simulink model "Idealized_BB_Model"  (R2017a)
settings: Solver=VariableStepDiscrete  StartTime=0.0  StopTime=inf  FixedStep=1/(PSF_SampPerSym*Rsymbol*2)  RelTol=1e-3  EnableMultiTasking=on
PreLoadFcn:
  | %Rates
  | BitRate=(250)*1e3;
  | ChipRate=2e6;
  | SymRate=ChipRate/2;
  | RX_ChipDelay=6;
  | 
  | %Pulse shaping filter
  | OS=32;
  | 
  | Pin=-40;
  | 
  | Gain=45;
  | NF=9;
  | 
  | fc_RF=2450e6;
InitFcn:
  | x=linspace(0,1,OS);
  | weights=sin(pi*x);
libraries: dspmlti4 x2, dspmathops x2, commdigbbndpm3 x2, dspstat3 x2, commrandsrc2 x1, commseqgen2 x1, commfilt2 x1, commsink2 x1, rfmathmodels1 x1, simulink x1
settings Model: Creator=The MathWorks Inc.  LastModifiedBy=gzucchel
settings DataIOCC: LimitDataPoints=on  SaveFormat=Array  SignalLoggingSaveFormat=ModelDataLogs  SaveOutput=off  SignalLogging=off  DSMLogging=off  SaveTime=off
settings OptimizationCC: ExpressionDepthLimit=2147483647  LifeSpan=inf
settings DebuggingCC: UnderspecifiedInitializationDetection=Classic  MergeDetectMultiDrivingBlocksExec=none  SolverPrmCheckMsg=warning  FcnCallInpInsideContextMsg=warning  StateNameClashWarn=warning  SFUnexpectedBacktrackingDiag=warning  SFNoUnconditionalDefaultTransitionDiag=warning  SFExecutionAtInitializationDiag=none
settings HardwareCC: ProdBitPerPointer=32  ProdBitPerSizeT=32  ProdBitPerPtrDiffT=32  ProdLargestAtomicFloat=None  ProdIntDivRoundTo=Undefined  ProdEndianess=Unspecified  ProdWordSize=32  ProdHWDeviceType=32-bit Generic
settings ModelReferenceCC: PropagateSignalLabelsOutOfModel=off
settings GRTTargetCC: TargetLangStandard=C89/C90 (ANSI)  GeneratePreprocessorConditionals=Disable all  CombineOutputUpdateFcns=off  GRTInterface=on
settings ConfigComp: CovMetricSettings=dw  CovHtmlReporting=on  CovSaveCumulativeToWorkspaceVar=on  CovSaveSingleToWorkspaceVar=on  CovExternalEMLEnable=off  CovSFcnEnable=off
settings SimscapeCC: SimscapeNormalizeSystem=off  SimscapeNominalValues="[{\"value\":\"10\",\"unit\":\"V\"},{\"value\":\"1\",\"unit\":\"A\"},{\"value\":\"10\",\"unit\":\"N*m\"},{\"value\":\"10\",\"unit\":\"bar\"},{\"value\":\"100\",\"unit\":\"kJ/kg\"},{\"value\":\"1\",\"unit\":\"kW\"},{\"value\":\"300\",\"unit\":\"K\"},{\"value\":\"100\",\"unit\":\"cm^3/s\"},{\"value\":\"1\",\"unit\":\"kN\"},{\"value\":\"1\",\"unit\":\"g/cm^3\"},{\"value\":\"1\",\"unit\":\"l\"},{\"value\":\"1\",\"unit\":\"cm^2\"},{\"value\":\"60\",\"unit\":\"Hz\"}]"
settings ConfigurationSet: Description=SimMechanics 2G

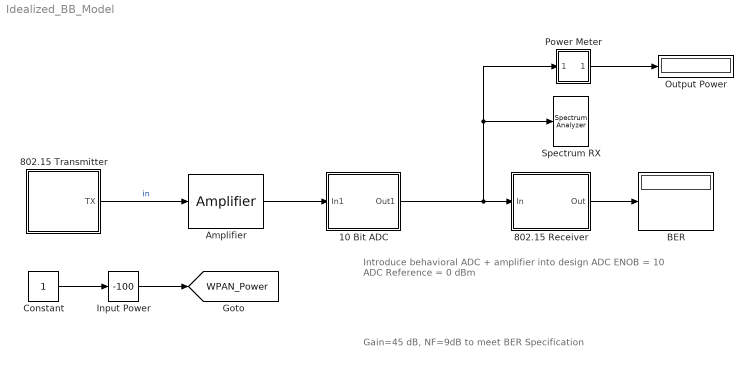
== system Idealized_BB_Model ==
  note: Introduce behavioral ADC + amplifier into design
      | ADC ENOB = 10
      | ADC Reference = 0 dBm
  note: Gain=45 dB, NF=9dB to meet BER Specification
  10 Bit ADC : Subsystem  mask{FS_P_dBm=0, Rnorm=1, N=10, Sample_Rate=0.0}
      mask prompts: FS_P_dBm "Full Scale Power"; Rnorm "Normalization Resistance"; Sample_Rate "Sample Rate (-1 for inherited)"
      mask init:
      | %LSB=FS_V/(2^(N-1));
      | %MAX=FS_V-LSB;
      | %MIN=-FS_V+LSB;
      | LSB=sqrt(2*Rnorm)*sqrt(1e-3)*sqrt(10^(FS_P_dBm/10))/(2^(N-1));
      | MAXp=sqrt(2*Rnorm)*sqrt(1e-3)*sqrt(10^(FS_P_dBm/10))-LSB;
      | MINp=-sqrt(2*Rnorm)*sqrt(1e-3)*sqrt(10^(FS_P_dBm/10))+LSB;
  802.15 Transmitter : Subsystem
  802.15 Receiver : Subsystem
  Amplifier : rfmathmodels1/Amplifier  model_select=Linear  linGaindB=Gain  GindB=0  iip3=30  am2pm=10  PwrAMPMStart=10  PwrAMPMEnd=inf  amam=[2.1587 1.1517]  ampm=[4.0033 9.1040]  x=[8.1081 1.5413 6.5202 -0.0718]  y=[4.6645 2.0965 10.88 -0.003]  p=0.5  GoutdB=0  vsat=1  method_select=Noise figure  ntemp=290  nfigure=NF  nfactor=0  seed=67987
      settings: SourceProductName=RF Toolbox  SourceProductBaseCode=RF
  BER : Display
  Constant : Constant
  Input Power : simulink/Math Operations/Slider Gain  gain=-100  low=-120  high=-30
  Output Power : Display
  Power Meter : Subsystem  mask{R=1, PB=off, buffer_sz=32*32}
      mask prompts: R "Resistance"; PB "Passband Power (Divide by 2)"; buffer_sz "Buffer Size"
  Spectrum RX : SpectrumAnalyzer
  tag scope: WPAN_Power=global
  wires:
  802.15 Receiver/1(Out) -> BER/1
  802.15 Transmitter/1(TX) -> Amplifier/1  "in"
  Power Meter/1(Power) -> Output Power/1
  Amplifier/1 -> 10 Bit ADC/1(In1)
  10 Bit ADC/1(Out1) -> Power Meter/1(In), Spectrum RX/1, 802.15 Receiver/1(In)
  Input Power/1 -> [WPAN_Power]
  Constant/1 -> Input Power/1

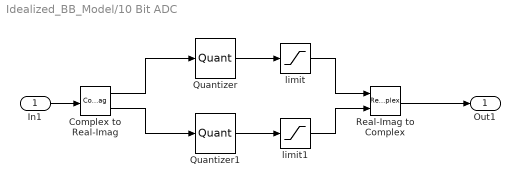
== system Idealized_BB_Model/10 Bit ADC ==
  In1 : Inport
  Complex to Real-Imag : ComplexToRealImag
  Quantizer : Quantizer  QuantizationInterval=LSB
  Quantizer1 : Quantizer  QuantizationInterval=LSB
  Real-Imag to Complex : RealImagToComplex
  limit : Saturate  UpperLimit=MAXp  LowerLimit=MINp
  limit1 : Saturate  UpperLimit=MAXp  LowerLimit=MINp
  Out1 : Outport
  wires:
  Quantizer/1 -> limit/1
  In1/1 -> Complex to Real-Imag/1
  Complex to Real-Imag/1 -> Quantizer/1
  Quantizer1/1 -> limit1/1
  Complex to Real-Imag/2 -> Quantizer1/1
  limit/1 -> Real-Imag to Complex/1
  limit1/1 -> Real-Imag to Complex/2
  Real-Imag to Complex/1 -> Out1/1

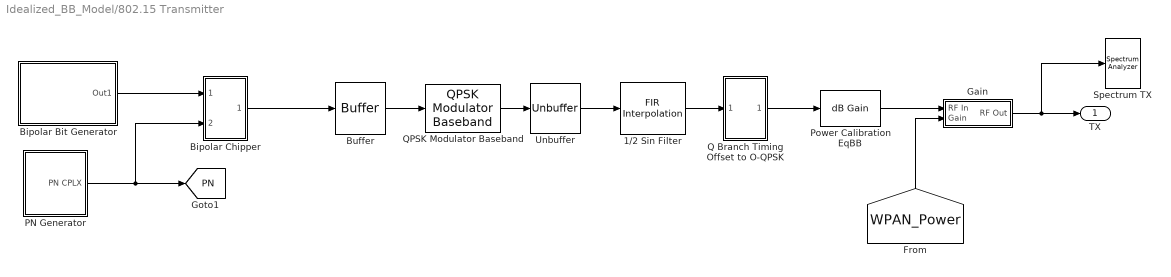
== system Idealized_BB_Model/802.15 Transmitter ==
  1/2 Sin Filter : dspmlti4/FIR Interpolation  FilterSource=Dialog parameters  h=weights  L=OS  FilterObject=Hm_firinterp  framing=Allow multirate processing  outputBufInitCond=0  roundingMode=Floor  overflowMode=off  firstCoeffDataTypeStr=Inherit: Same word length as input  firstCoeffMin=[]  firstCoeffMax=[]  firstCoeffLastDataTypeStr=Inherit: Same word length as input  outputDataTypeStr=Inherit: Same as accumulator  outputMin=[]  outputMax=[]  outputLastDataTypeStr=Inherit: Same as accumulator
      settings: SourceProductName=DSP System Toolbox
  Bipolar Chipper : Subsystem
  Bipolar Bit Generator : Subsystem
  Buffer : Buffer  N=2
  Gain : Subsystem
  PN Generator : Subsystem
  Power Calibration EqBB : dspmathops/dB Gain  dB=-26.8  intype=Amplitude
      settings: SourceProductName=DSP System Toolbox  SourceProductBaseCode=DS
  Q Branch Timing Offset to O-QPSK : Subsystem
  QPSK Modulator Baseband : commdigbbndpm3/QPSK Modulator Baseband  InType=Bit  Enc=Gray  Ph=pi/4  outDtype=double  outWordLen=16  outUDDataType=sfix(16)  outFracLenMode=Best precision  outFracLen=15  outDataTypeStr=double  outLastDataTypeStr=double
  Spectrum TX : SpectrumAnalyzer
  Unbuffer : Unbuffer
  TX : Outport
  tag scope: PN=global
  wires:
  QPSK Modulator Baseband/1 -> Unbuffer/1
  1/2 Sin Filter/1 -> Q Branch Timing Offset to O-QPSK/1(In1)
  PN Generator/1(PN CPLX) -> Bipolar Chipper/2(In2), [PN]
  Bipolar Bit Generator/1(Out1) -> Bipolar Chipper/1(In1)
  Bipolar Chipper/1(Out1) -> Buffer/1
  Buffer/1 -> QPSK Modulator Baseband/1
  Unbuffer/1 -> 1/2 Sin Filter/1
  [WPAN_Power] -> Gain/2(Gain)
  Gain/1(RF Out) -> TX/1, Spectrum TX/1
  Q Branch Timing Offset to O-QPSK/1(Out1) -> Power Calibration EqBB/1
  Power Calibration EqBB/1 -> Gain/1(RF In)

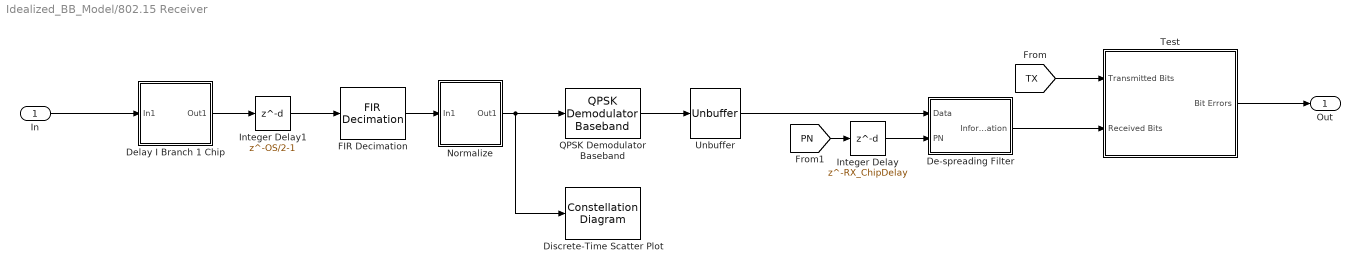
== system Idealized_BB_Model/802.15 Receiver ==
  In : Inport
  De-spreading Filter : Subsystem
  Delay I Branch 1 Chip : Subsystem
  Discrete-Time Scatter Plot : ConstellationDiagram  Tag=ScatterPlot
  FIR Decimation : dspmlti4/FIR Decimation  FilterSource=Dialog parameters  h=fliplr(conj(weights))  D=OS  filtStruct=Direct form  FilterObject=Hm_firdecim  InputProcessing=Columns as channels (frame based)  framing=Allow multirate processing  inputOffset=0  outputBufInitCond=0  roundingMode=Floor  overflowMode=off  firstCoeffDataTypeStr=Inherit: Same word length as input  firstCoeffMin=[]  firstCoeffMax=[]  firstCoeffLastDataTypeStr=Inherit: Same word length as input  outputDataTypeStr=Inherit: Same as accumulator  outputMin=[]  outputMax=[]  outputLastDataTypeStr=Inherit: Same as accumulator
  Integer Delay : Delay  DelayLength=RX_ChipDelay
  Integer Delay1 : Delay  DelayLength=OS/2-1
  Normalize : Subsystem
  QPSK Demodulator Baseband : commdigbbndpm3/QPSK Demodulator Baseband  OutType=Bit  DecType=Hard decision  VarSource=Dialog  Variance=1  Dec=Gray  Ph=pi/4  outDtype1=Inherit via internal rule  outDtype2=Inherit via internal rule  derotateFactorWordLen=16  derotateFactorDataTypeStr=Inherit: Same word length as input  derotateFactorLastDataTypeStr=Inherit: Same word length as input
  Test : Subsystem
  Unbuffer : Unbuffer
  Out : Outport
  wires:
  De-spreading Filter/1(Information) -> Test/2(Received Bits)
  Integer Delay/1 -> De-spreading Filter/2(PN)
  [PN] -> Integer Delay/1
  Unbuffer/1 -> De-spreading Filter/1(Data)
  Normalize/1(Out1) -> QPSK Demodulator Baseband/1, Discrete-Time Scatter Plot/1
  Integer Delay1/1 -> FIR Decimation/1
  FIR Decimation/1 -> Normalize/1(In1)
  QPSK Demodulator Baseband/1 -> Unbuffer/1
  In/1 -> Delay I Branch 1 Chip/1(In1)
  Delay I Branch 1 Chip/1(Out1) -> Integer Delay1/1
  Test/1(Bit Errors) -> Out/1
  [TX] -> Test/1(Transmitted Bits)

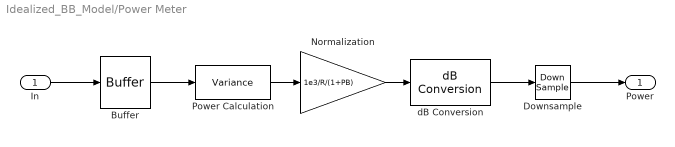
== system Idealized_BB_Model/Power Meter ==
  In : Inport
  Buffer : Buffer  N=buffer_sz
  Downsample : DownSample  N=100  RateOptions=Allow multirate processing
  Normalization : Gain  Gain=1e3/R/(1+PB)
  Power Calculation : dspstat3/Variance  run=off  reset_popup=None  InputProcessing=Columns as channels (frame based)  directionMode=Each column  dimension=1  roiEnable=off  roiType=Rectangles  roiPortion=Entire ROI  roiOutput=Individual statistics for each ROI  roiFlag=off  roundingMode=Floor  overflowMode=off
      settings: SourceProductName=DSP System Toolbox
  dB Conversion : dspmathops/dB Conversion  dBtype=dB  intype=Power  R=1  fuzz=on
      settings: SourceProductName=DSP System Toolbox
  Power : Outport
  wires:
  dB Conversion/1 -> Downsample/1
  Buffer/1 -> Power Calculation/1
  In/1 -> Buffer/1
  Normalization/1 -> dB Conversion/1
  Power Calculation/1 -> Normalization/1
  Downsample/1 -> Power/1

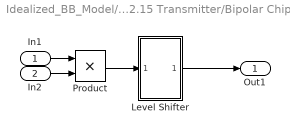
== system Idealized_BB_Model/802.15 Transmitter/Bipolar Chipper ==
  In1 : Inport
  In2 : Inport  Port=2
  Level Shifter : Subsystem
  Product : Product  RndMeth=Zero
  Out1 : Outport
  wires:
  In2/1 -> Product/2
  Level Shifter/1(Out1) -> Out1/1
  In1/1 -> Product/1
  Product/1 -> Level Shifter/1(In1)

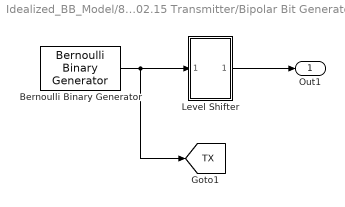
== system Idealized_BB_Model/802.15 Transmitter/Bipolar Bit Generator ==
  Bernoulli Binary Generator : commrandsrc2/Bernoulli Binary Generator  P=0.5  seed=61  Ts=1/BitRate  frameBased=off  sampPerFrame=1  orient=off  outDataType=double
  Level Shifter : Subsystem
  Out1 : Outport
  tag scope: TX=global
  wires:
  Level Shifter/1(Out1) -> Out1/1
  Bernoulli Binary Generator/1 -> [TX], Level Shifter/1(In1)

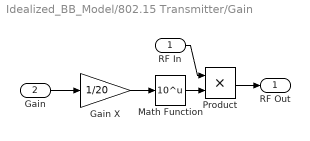
== system Idealized_BB_Model/802.15 Transmitter/Gain ==
  RF In : Inport
  Gain : Inport  Port=2
  Gain X : Gain  Gain=1/20
  Math Function : Math  Operator=10^u  SaturateOnIntegerOverflow=on
  Product : Product  RndMeth=Zero
  RF Out : Outport
  wires:
  Gain/1 -> Gain X/1
  Product/1 -> RF Out/1
  RF In/1 -> Product/1
  Math Function/1 -> Product/2
  Gain X/1 -> Math Function/1

== system Idealized_BB_Model/802.15 Transmitter/PN Generator ==
  Level Shifter : Subsystem
  Scrambling code : commseqgen2/PN Sequence Generator  poly=[0 -7 -10]  ini_sta=[1 0 0 0 0 0 0 0 0 0]  outBitMaskSource=Dialog parameter  shift=0  outVarSiz=off  maxOutSizeMode=Dialog parameter  maxOutSize=[10 1]  Ts=1/ChipRate  frameBased=off  sampPerFrame=1  reset=off  bitPackedOutputs=off  outDataType=double  numPackedBits=8  bitPackDataSigned=off  bitPackedOutDType=double
  PN CPLX : Outport
  wires:
  Level Shifter/1(Out1) -> PN CPLX/1
  Scrambling code/1 -> Level Shifter/1(In1)

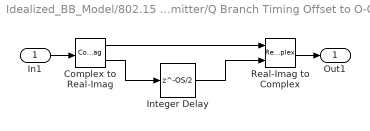
== system Idealized_BB_Model/802.15 Transmitter/Q Branch Timing Offset to O-QPSK ==
  In1 : Inport
  Complex to Real-Imag : ComplexToRealImag
  Integer Delay : Delay  DelayLength=OS/2
  Real-Imag to Complex : RealImagToComplex
  Out1 : Outport
  wires:
  Real-Imag to Complex/1 -> Out1/1
  In1/1 -> Complex to Real-Imag/1
  Complex to Real-Imag/1 -> Real-Imag to Complex/1
  Integer Delay/1 -> Real-Imag to Complex/2
  Complex to Real-Imag/2 -> Integer Delay/1

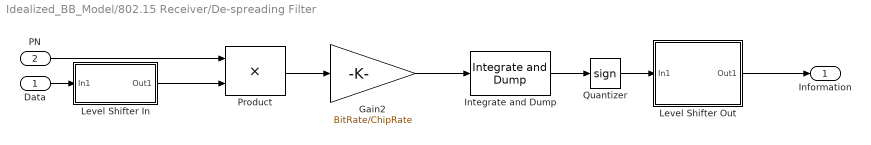
== system Idealized_BB_Model/802.15 Receiver/De-spreading Filter ==
  Data : Inport
  PN : Inport  Port=2
  Gain2 : Gain  Gain=BitRate/ChipRate  SaturateOnIntegerOverflow=on  OutDataTypeStr=Inherit: Same as input  ParamDataTypeStr=Inherit: Same as input
  Integrate and Dump : commfilt2/Integrate and Dump  obssamples=ChipRate/BitRate  offsetsamples=RX_ChipDelay  nodump=off  roundingMode=Floor  overflowMode=off  outputDataTypeStr=Inherit: Same as accumulator  outputLastDataTypeStr=Inherit: Same as accumulator
      settings: SourceProductName=Communications System Toolbox
  Level Shifter In : Subsystem
  Level Shifter Out : Subsystem
  Product : Product  RndMeth=Zero
  Quantizer : Signum
  Information : Outport
  wires:
  Quantizer/1 -> Level Shifter Out/1(In1)
  PN/1 -> Product/1
  Integrate and Dump/1 -> Quantizer/1
  Level Shifter In/1(Out1) -> Product/2
  Product/1 -> Gain2/1
  Gain2/1 -> Integrate and Dump/1
  Level Shifter Out/1(Out1) -> Information/1
  Data/1 -> Level Shifter In/1(In1)

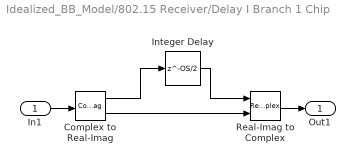
== system Idealized_BB_Model/802.15 Receiver/Delay I Branch 1 Chip ==
  In1 : Inport
  Complex to Real-Imag : ComplexToRealImag
  Integer Delay : Delay  DelayLength=OS/2
  Real-Imag to Complex : RealImagToComplex
  Out1 : Outport
  wires:
  Real-Imag to Complex/1 -> Out1/1
  In1/1 -> Complex to Real-Imag/1
  Complex to Real-Imag/2 -> Real-Imag to Complex/2
  Integer Delay/1 -> Real-Imag to Complex/1
  Complex to Real-Imag/1 -> Integer Delay/1

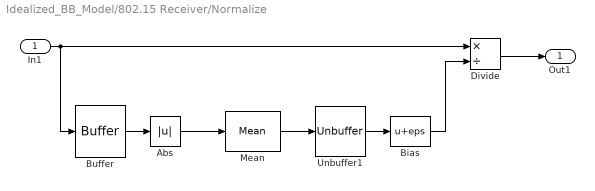
== system Idealized_BB_Model/802.15 Receiver/Normalize ==
  In1 : Inport
  Abs : Abs
  Bias : Bias  Bias=eps
  Buffer : Buffer
  Divide : Product  Inputs=*/
  Mean : dspstat3/Mean  run=off  reset_popup=None  InputProcessing=Columns as channels (frame based)  directionMode=Each column  dimension=1  roiEnable=off  roiType=Rectangles  roiPortion=Entire ROI  roiOutput=Individual statistics for each ROI  roiFlag=off  outputDataTypeStr=Inherit: Same as accumulator  outputLastDataTypeStr=Inherit: Same as accumulator  outputMin=[]  outputMax=[]  roundingMode=Floor  overflowMode=off
  Unbuffer1 : Unbuffer
  Out1 : Outport
  wires:
  Bias/1 -> Divide/2
  Unbuffer1/1 -> Bias/1
  Divide/1 -> Out1/1
  In1/1 -> Divide/1, Buffer/1
  Mean/1 -> Unbuffer1/1
  Abs/1 -> Mean/1
  Buffer/1 -> Abs/1

== system Idealized_BB_Model/802.15 Receiver/Test ==
  Transmitted Bits : Inport
  Received Bits : Inport  Port=2
  Error Rate Calculation : commsink2/Error Rate Calculation  N=2  st_delay=2  cp_mode=Entire frame  subframe=[]  PMode=Port  WsName=ErrorVec  RsMode2=off  stop=off  numErr=inf  maxBits=20000
  Bit Errors : Outport
  wires:
  Received Bits/1 -> Error Rate Calculation/2
  Error Rate Calculation/1 -> Bit Errors/1
  Transmitted Bits/1 -> Error Rate Calculation/1

== system Idealized_BB_Model/802.15 Transmitter/Bipolar Chipper/Level Shifter ==
  In1 : Inport
  Bias : Bias  Bias=1
  Gain : Gain  Gain=0.5
  Out1 : Outport
  wires:
  Gain/1 -> Out1/1
  In1/1 -> Bias/1
  Bias/1 -> Gain/1

== system Idealized_BB_Model/802.15 Transmitter/Bipolar Bit Generator/Level Shifter ==
  In1 : Inport
  Bias : Bias  Bias=-1
  Gain : Gain  Gain=2
  Out1 : Outport
  wires:
  Bias/1 -> Out1/1
  In1/1 -> Gain/1
  Gain/1 -> Bias/1

== system Idealized_BB_Model/802.15 Transmitter/PN Generator/Level Shifter ==
  In1 : Inport
  Bias : Bias  Bias=-1
  Gain : Gain  Gain=2
  Out1 : Outport
  wires:
  In1/1 -> Gain/1
  Bias/1 -> Out1/1
  Gain/1 -> Bias/1

== system Idealized_BB_Model/802.15 Receiver/De-spreading Filter/Level Shifter In ==
  In1 : Inport
  Bias : Bias  Bias=-1
  Gain : Gain  Gain=2
  Out1 : Outport
  wires:
  In1/1 -> Gain/1
  Bias/1 -> Out1/1
  Gain/1 -> Bias/1

== system Idealized_BB_Model/802.15 Receiver/De-spreading Filter/Level Shifter Out ==
  In1 : Inport
  Bias1 : Bias  Bias=1
  Gain1 : Gain  Gain=0.5
  Out1 : Outport
  wires:
  Gain1/1 -> Out1/1
  In1/1 -> Bias1/1
  Bias1/1 -> Gain1/1
